simulink model "Q1a2017"  (R2017b)
settings: Solver=VariableStepAuto  StartTime=0.0  StopTime=10.0  RelTol=1e-3
settings Model: Creator=Kasra  LastModifiedBy=Kasra

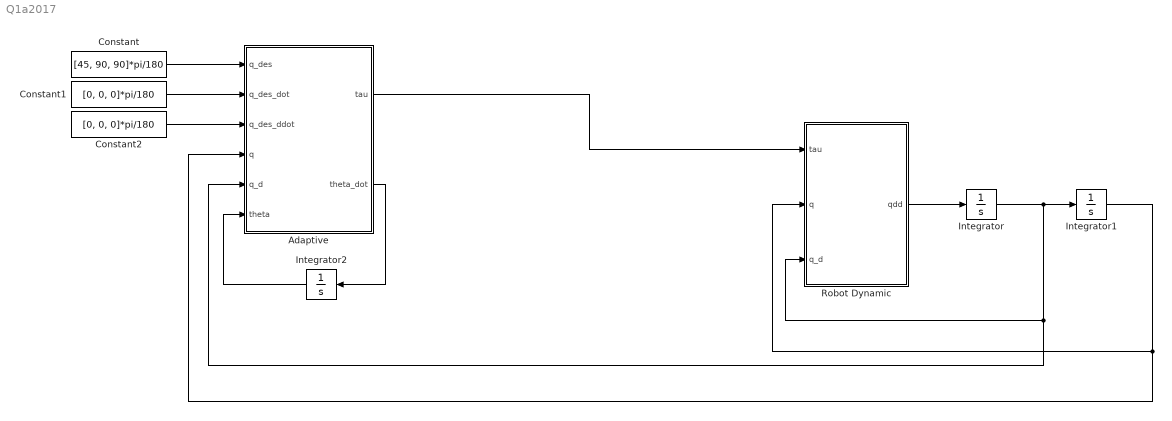
== system Q1a2017 ==
  Adaptive : MATLAB Function  TreatAsAtomicUnit=on
  Constant : Constant  Value=[45, 90, 90]*pi/180
  Constant1 : Constant  Value=[0, 0, 0]*pi/180
  Constant2 : Constant  Value=[0, 0, 0]*pi/180
  Integrator : Integrator  InitialCondition=[0,0,0]
  Integrator1 : Integrator  InitialCondition=[0,0,0]
  Integrator2 : Integrator  InitialCondition=[0,0,0,0]
  Robot Dynamic : MATLAB Function  TreatAsAtomicUnit=on
  wires:
  Integrator/1 -> Robot Dynamic/3(q_d), Adaptive/5(q_d), Integrator1/1
  Robot Dynamic/1(qdd) -> Integrator/1
  Integrator1/1 -> Robot Dynamic/2(q), Adaptive/4(q)
  Adaptive/2(theta_dot) -> Integrator2/1
  Integrator2/1 -> Adaptive/6(theta)
  Adaptive/1(tau) -> Robot Dynamic/1(tau)
  Constant/1 -> Adaptive/1(q_des)
  Constant1/1 -> Adaptive/2(q_des_dot)
  Constant2/1 -> Adaptive/3(q_des_ddot)

== matlab function Q1a2017/Adaptive ==
  data: q_des input; tau output; q_des_dot input; q_des_ddot input; q input; q_d input; theta input; theta_dot output
function [tau, theta_dot] = fcn(q_des, q_des_dot, q_des_ddot, q, q_d, theta)


q_tilda = q - q_des;
gamma = 2;
v = q_des_dot - gamma*q_tilda;
q_tilda_dot = q_d - q_des_dot;
v_d = q_des_ddot - gamma * q_tilda_dot;
r = q_d - v;


g=9.8;

y = [v_d(1), v_d(2), (2*v_d(1)+v_d(2))*cos(q(1))-(q_d(2)*v(2)+q_d(1)*v(2)+v(1)*q_d(2)) 0;0, (v_d(1)+v_d(2)), (v_d(1)*cos(q(2))+(v_d(2)^(2))*sin(q(2))), 0;0, 0, 0, v_d(3)-g];
gam = 0.1;
theta_dot = -pinv(gam)*y'*r;
k = 5*eye(3);
tau = y*theta+k*r;

%q1 = q(1);
%q2 = q(2);
%q3 = q(3);

%q1d = q_d(1);
%q2d = q_d(2);
%q3d = q_d(3);

%g = 9.81;

%%%%%%%%%%

%v = q_des_d - gamma * q_tilde;
%v_d = q_des_dd - gamma * q_tilde_d;
%r = qd - v;

%Y1 = [v_d(1), v_d(2), (2 * v_d(1) + v_d(2))*cos(q2) - (v(2) * q2d + 2*v(1)*q2d)*sin(q2), 0];
%Y2 = [0, v_d(1)+v_d(2), v_d(1)*cos(q2)+v_d(2)*q1d*sin(q2), 0]
%Y3 = [0, 0, 0, v_d(3) - g]

%Y = blkdiag(Y1, Y2, Y3);

%gam = 0.1;
%theta_dot = -pinv(gam)*Y'*r;

%K = 5*eye(3);
%tau = Y*theta-K*r;

== matlab function Q1a2017/Robot Dynamic ==
  data: tau input; qdd output; q input; q_d input
function qdd = fcn(tau, q, q_d)

m1=12;
m2=6;
m3=6;
I1 = 0.36;
I2 = 0.36;
a1 = 0.6;
a2 = 0.4;
lc1 = 0.3;
lc2 = 0.2;
g = 9.8;


M11 = m1*lc1^(2)+(m2*(a1^(2)+lc2^(2)+2*a1*lc1*cos(q(2))))+m3*(a1^(2)+a2^(2)+2*a1*a2*cos(q(2)))+I1+I2;
M12 = m2*lc2*(lc2+a1*cos(q(2)))+m3*(a1*a2*cos(q(2))+a2^(2))+I2;
M21 = M12;
M33 = m3;
M22 = m2*lc2^(2)+m3*a2^(2)+I2;
M=[M11 M12 0;M21 M22 0;0 0 M33];
h=(m2*a1*lc2+m3*a2*a1)*sin(q(2));
C=[-2*h*q_d(1) -h*q_d(2) 0;h*q_d(1) 0 0;0 0 0];
G=[0;0;-m3*g];
q_dd = pinv(M)*(tau - C*q_d - G);
